simulink model "planta"  (R2020b)
settings: Solver=VariableStepAuto  StartTime=0.0  StopTime=10.0  RelTol=1e-3
settings Model: Creator=Advance  LastModifiedBy=Advance

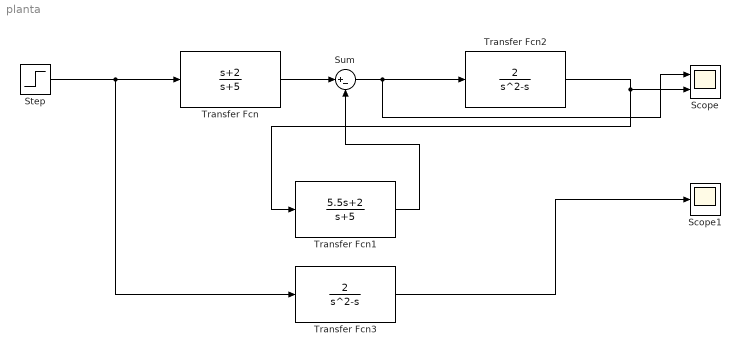
== system planta ==
  Scope : Scope  NumInputPorts=2
  Scope1 : Scope
  Step : Step  Time=0  After=100  SampleTime=0
  Sum : Sum  Inputs=|+-
  Transfer Fcn : TransferFcn  Numerator=[1 2]  Denominator=[1 5]
  Transfer Fcn1 : TransferFcn  Numerator=[5.5 2]  Denominator="[1  5]"
  Transfer Fcn2 : TransferFcn  Numerator=[ 2]  Denominator="[1  -1 0]"
  Transfer Fcn3 : TransferFcn  Numerator=[ 2]  Denominator="[1  -1 0]"
  wires:
  Step/1 -> Transfer Fcn3/1, Transfer Fcn/1
  Transfer Fcn/1 -> Sum/1
  Transfer Fcn1/1 -> Sum/2
  Transfer Fcn2/1 -> Transfer Fcn1/1, Scope/2
  Sum/1 -> Scope/1, Transfer Fcn2/1
  Transfer Fcn3/1 -> Scope1/1
